simulink model "quadcopter_swarm_Perron_quaternion"  (R2023b)
settings: Solver=ode3  StartTime=0  StopTime=inf  FixedStep=0.005  RelTol=1e-3  EnableMultiTasking=on
values from neighbouring files (symbols this model uses):
  epsilon = 0.24975    [1nrx_dot.mat]    (also in 1nrxdrones_dot.mat; collision_avoidance_POS.mat; collision_avoidance_headonfix_POS.mat; collision_test.mat)
  F_e_g = [0 0 39.28]    [1nrx_dot.mat]    (also in 1nrxdrones_dot.mat; collision_avoidance_POS.mat; collision_avoidance_headonfix_POS.mat; collision_test.mat)
  g = 9.82    [1nrx_dot.mat]    (also in 1nrxdrones_dot.mat; collision_avoidance_POS.mat; collision_avoidance_headonfix_POS.mat; collision_test.mat)
  I_C = [0.5  0  0; 0  0.5  0; 0  0  1]    [1nrx_dot.mat]    (also in 1nrxdrones_dot.mat; collision_avoidance_POS.mat; collision_avoidance_headonfix_POS.mat; collision_test.mat)
  L = [4 -1 -1 -1 -1 0 -1 4 -1 -1 -1 0 ... (36 elements, 6x6)]    [1nrx_dot.mat]    (also in 1nrxdrones_dot.mat; collision_avoidance_POS.mat; collision_avoidance_headonfix_POS.mat; collision_test.mat)
  m = 4    [1nrx_dot.mat]    (also in 1nrxdrones_dot.mat; collision_avoidance_POS.mat; collision_avoidance_headonfix_POS.mat; collision_test.mat)
  M_RB = [4 0 0 0 0 0 0 4 0 0 0 0 ... (36 elements, 6x6)]    [1nrx_dot.mat]    (also in 1nrxdrones_dot.mat; collision_avoidance_POS.mat; collision_avoidance_headonfix_POS.mat; collision_test.mat)
  p_0 = [5  10; 5  -5; -8  5; 5  -13; 8  8; 0  0]    [1nrx_dot.mat]    (also in 1nrxdrones_dot.mat; collision_avoidance_POS.mat; collision_avoidance_headonfix_POS.mat; collision_test.mat)
  p_d = [1  0; 4  0; -2  0; 7  0; 9  0; 0  0]    [1nrx_dot.mat]    (also in 1nrxdrones_dot.mat; collision_avoidance_POS.mat; collision_avoidance_headonfix_POS.mat; collision_test.mat)
  V = [1 2 3 4 5 6]    [1nrx_dot.mat]    (also in 1nrxdrones_dot.mat; collision_avoidance_POS.mat; collision_avoidance_headonfix_POS.mat; collision_test.mat)
undefined symbols (not defined in the file or in its folder): PID_angle_max, PID_inner_max, PID_outer_max, PID_thrust_max
libraries: slpidlib x24, simulink_extras x20, dspsigops x15, sharedtransform x13, aerolibutil x11, dspindex x4, sharedutil x1, vrlib x1
(part 1 of 5)
settings Model: Creator=The MathWorks, Inc.  LastModifiedBy=frank
settings SolverCC: AlgebraicLoopSolver=TrustRegion
settings DataIOCC: LimitDataPoints=on  SaveFormat=Array  SaveOutput=off  SignalLogging=off  DSMLogging=off  SaveTime=off  ReturnWorkspaceOutputs=off
settings OptimizationCC: BlockReduction=off  BufferReuse=off  LifeSpan=inf
settings DebuggingCC: AlgebraicLoopMsg=none  ParameterPrecisionLossMsg=none  AllowSymbolicDim=off  PregeneratedLibrarySubsystemCodeDiagnostic=none  SFUnexpectedBacktrackingDiag=warning  SFNoUnconditionalDefaultTransitionDiag=warning  SFExecutionAtInitializationDiag=none  ArithmeticOperatorsInVariantConditions=warning
settings HardwareCC: ProdBitPerPointer=32  ProdBitPerSizeT=32  ProdBitPerPtrDiffT=32  ProdLargestAtomicFloat=None  ProdIntDivRoundTo=Undefined  ProdEndianess=Unspecified  ProdWordSize=32  ProdHWDeviceType=32-bit Generic
settings ModelReferenceCC: EnableRefExpFcnMdlSchedulingChecks=on  PropagateSignalLabelsOutOfModel=off
settings SFSimCC: SimUseLocalCustomCode=off  CustomCodeUndefinedFunction=UseInterfaceOnly
settings RTWCC: RTWUseLocalCustomCode=off  DLArmComputeVersion=19.05
settings CodeAppCC: StateflowObjectComments=on
settings GRTTargetCC: TargetLangStandard=C89/C90 (ANSI)
settings ConfigComp: CovMetricSettings=dw  CovSaveCumulativeToWorkspaceVar=on  CovSaveSingleToWorkspaceVar=on  CovExternalEMLEnable=off  CovSFcnEnable=off

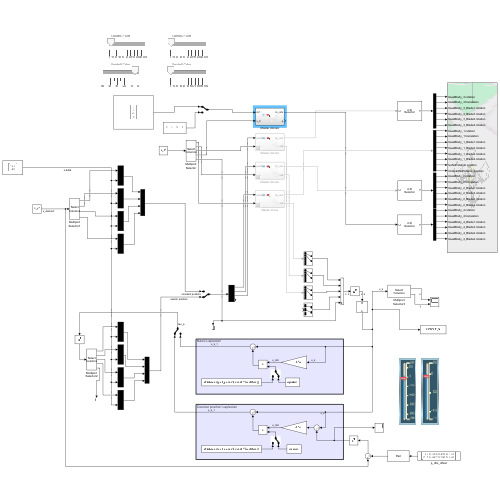
[thumbnail: Simulink's stored preview of the top-level diagram]
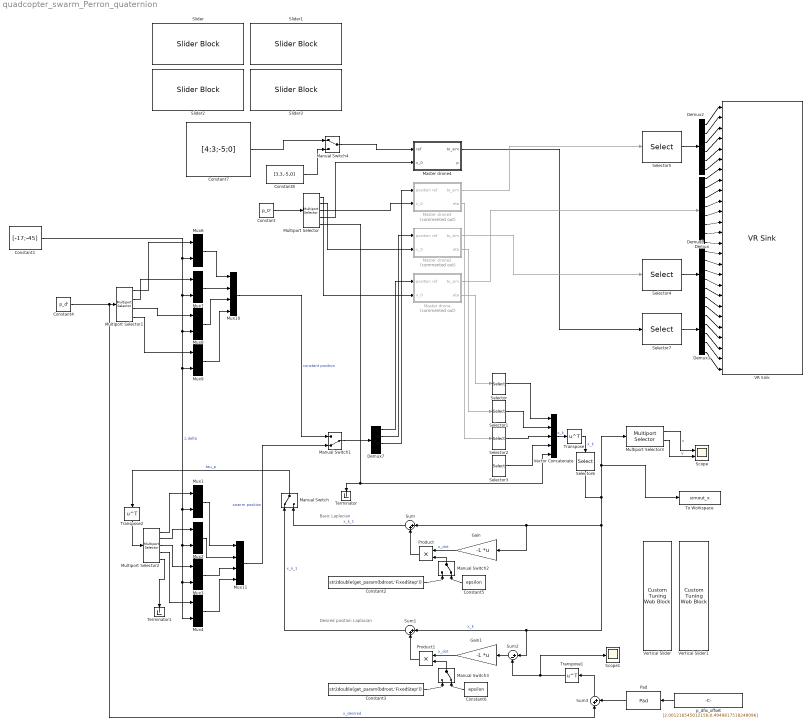
== system quadcopter_swarm_Perron_quaternion ==
  note: Basic Laplacian
  note: Desired position Laplacian
  Constant : Constant  Value=p_0'
  Constant1 : Constant  Value=[-17;-45]  VectorParams1D=off
  Constant2 : Constant  Value=str2double(get_param(bdroot,'FixedStep'))
  Constant3 : Constant  Value=str2double(get_param(bdroot,'FixedStep'))
  Constant4 : Constant  Value=p_d'
  Constant5 : Constant  Value=epsilon
  Constant6 : Constant  Value=epsilon
  Constant7 : Constant  Value=[4;3;-5;0]  VectorParams1D=off
  Constant8 : Constant  Value=[3,3,-5,0]
  Demux : Demux  Outputs=8
  Demux1 : Demux  Outputs=6
  Demux2 : Demux  Outputs=6
  Demux3 : Demux  Outputs=6
  Demux7 : Demux
  Gain : Gain  Gain=-L  Multiplication=Matrix(K*u)
  Gain1 : Gain  Gain=-L  Multiplication=Matrix(K*u)
  Manual Switch : ManualSwitch
  Manual Switch1 : ManualSwitch  CurrentSetting=0
  Manual Switch2 : ManualSwitch  CurrentSetting=0
  Manual Switch3 : ManualSwitch  CurrentSetting=0
  Manual Switch4 : ManualSwitch
  Master drone : Subsystem  Commented=on
  Master drone2 : Subsystem  Commented=on
  Master drone3 : Subsystem  Commented=on
  Master drone4 : Subsystem
  Multiport Selector : dspindex/Multiport Selector  rowsOrCols=Columns  idxCellArray={1,2,3,4,5}  idxErrMode=Clip Index
      settings: LibrarySourceBlock=|
      | dsphdlsupportsigmgmt/Multiport
      | Selector
  Multiport Selector1 : dspindex/Multiport Selector  rowsOrCols=Columns  idxCellArray={1,2,3,4}  idxErrMode=Clip Index
      settings: LibrarySourceBlock=|
      | dsphdlsupportsigmgmt/Multiport
      | Selector
  Multiport Selector2 : dspindex/Multiport Selector  rowsOrCols=Columns  idxCellArray={1,2,3,4,5}  idxErrMode=Clip Index
      settings: LibrarySourceBlock=|
      | dsphdlsupportsigmgmt/Multiport
      | Selector
  Multiport Selector3 : dspindex/Multiport Selector  rowsOrCols=Columns  idxCellArray={1,2}  idxErrMode=Clip Index
      settings: LibrarySourceBlock=|
      | dsphdlsupportsigmgmt/Multiport
      | Selector
  Mux{1..4,6..9} (8 alike) : Mux  Inputs=2
  Mux10 : Mux
  Mux11 : Mux
  Pad : dspsigops/Pad  padAlong=Rows  dimsToPad=1  valSrc=Specify via dialog  padVal=0  spec=Output size  padNumOutRowsSpecMethod=User-specified  numOutRows=2  padNumOutColsSpecMethod=User-specified  numOutCols=size(p_d,1)  isVarDimsMode=off  padBeginning=0  padEnd=0  outSizeMode=User-specified  outSize=1  padSigAt=Beginning  trunc_flag=None  roundingMode=Floor  overflowMode=off  truncOrWrapMode=Truncate  wrap_flag=None
  Product : Product
  Product1 : Product
  Scope : Scope  NumInputPorts=2
  Scope1 : Scope
  Selector : Selector  InputPortWidth=6  IndexOptions=Index vector (dialog)  Indices=1:2  OutputSizes=1
  Selector1 : Selector  InputPortWidth=6  IndexOptions=Index vector (dialog)  Indices=1:2  OutputSizes=1
  Selector2 : Selector  InputPortWidth=6  IndexOptions=Index vector (dialog)  Indices=1:2  OutputSizes=1
  Selector3 : Selector  InputPortWidth=3  IndexOptions=Index vector (dialog)  Indices=1:2  OutputSizes=1
  Selector4 : Selector  NumberOfDimensions=2  InputPortWidth=8  IndexOptions=Index vector (dialog),Select all  Indices=1:23,1  OutputSizes=1,1
  Selector5 : Selector  NumberOfDimensions=2  InputPortWidth=8  IndexOptions=Index vector (dialog),Select all  Indices=1:23,1  OutputSizes=1,1
  Selector6 : Selector  NumberOfDimensions=2  InputPortWidth=3  IndexOptions=Index vector (dialog),Select all  Indices=V,1  OutputSizes=1,1
  Selector7 : Selector  NumberOfDimensions=2  InputPortWidth=8  IndexOptions=Index vector (dialog),Select all  Indices=1:23,1  OutputSizes=1,1
  Slider : SliderBlock
  Slider1 : SliderBlock
  Slider2 : SliderBlock  ScaleMin=-50  ScaleMax=0
  Slider3 : SliderBlock
  Sum : Sum  Inputs=|++
  Sum1 : Sum  Inputs=|++
  Sum2 : Sum  Inputs=|+-
  Sum3 : Sum  Inputs=|++
  Terminator : Terminator
  Terminator1 : Terminator
  To Workspace : ToWorkspace  VariableName=simout_x  SampleTime=-1
      settings: Save2DSignal=2-D array (concatenate along first dimension)
  Transpose : Math  Operator=transpose
  Transpose1 : Math  Operator=transpose
  Transpose2 : Math  Operator=transpose
  VR Sink : vrlib/VR Sink  InstantiateOnLoad=on  SampleTime=12*0.005  ViewEnable=on  RemoteChange=off  RemoteView=off  FieldsWritten=QuadBody_3.rotation.4.1.1.double#QuadBody_3.translation.3.1.1.double#QuadBody_3_Blade1.rotation.4.1.1.double#QuadBody_3_Blade3.rotation.4.1.1.double#QuadBody_3_Blade2.rotation.4.1.1.double#QuadBody_3_Blade4.rotation.4.1.1.double#QuadBody_1.rotation.4.1.1.double#QuadBody_1.translation.3.1.1.double#QuadBody_1_Blade1.rotation.4.1.1.double#QuadBody_1_Blade3.rotation.4.1.1.double#QuadBody_1_Blade2.rotation.4.1.1.double#QuadBody_1_Blade4.rotation.4.1.1.double#IsoNoRotation.position.3.1.1.double#OnQuadNoRotation.position.3.1.1.double#QuadBody_2.rotation.4.1.1.double#QuadBody_2.translation.3.1.1.double#QuadBody_2_Blade1.rotation.4.1.1.double#QuadBody_2_Blade3.rotation.4.1.1.double#QuadBody_2_Blade2.rotation.4.1.1.double#QuadBody_2_Blade4.rotation.4.1.1.double#QuadBody_4.rotation.4.1.1.double#QuadBody_4.translation.3.1.1.double#QuadBody_4_Blade1.rotation.4.1.1.double#QuadBody_4_Blade3.rotation.4.1.1.double#QuadBody_4_Blade2.rotation.4.1.1.double#QuadBody_4_Blade4.rotation.4.1.1.double  WorldFileName=Quadcopter_VR.wrl  AutoView=on  VideoDimensions=[]  AllowVariableSize=off  FigureProperties="{'Position', 'Name', 'Viewpoint', 'CameraBound', 'CameraDirection', 'CameraPosition', 'CameraUpVector', 'ZoomFactor', 'Antialiasing', 'Headlight', 'Lighting', 'NavPanel', 'Sound', 'StatusBar', 'Stereo3D', 'Stereo3DCameraOffset', 'Stereo3DHIT', 'ToolBar', 'Textures', 'Transparency', 'Triad', 'Wireframe', 'NavZones', 'NavMode', 'NavSpeed', 'CaptureFileFormat', 'CaptureFileName', 'Record2DCompressMethod', 'Record2DCompressQuality', 'Record2D', 'Record2DFileName', 'Record2DFPS'; [2.0000000000000000e+00   8.4000000000000000e+01   8.6000000000000000e+02   5.6400000000000000e+02], '', 'Quad 4', 'on', [0.0000000000000000e+00   0.0000000000000000e+00  -1.0000000000000000e+00], [0.0000000000000000e+00   0.0000000000000000e+00   0.0000000000000000e+00], [0.0000000000000000e+00   1.0000000000000000e+00   0.0000000000000000e+00], [1.0000000000000000e+00], 'on', 'on', 'on', 'halfbar', 'on', 'on', 'off', [1.0000000149011612e-01], [0.0000000000000000e+00], 'on', 'on', 'on', 'none', 'off', 'off', 'examine', 'normal', 'tif', '%f_anim_%n.tif', 'auto', [7.5000000000000000e+01], 'off', '%f_anim_%n.avi', 'auto'}"
  Vector Concatenate : Concatenate  NumInputs=5  Mode=Multidimensional array  ConcatenateDimension=2
  Vertical Slider : CustomTuningWebBlock  LabelPosition=Hide  ShowInitialText=on  Configuration="{\"components\":[{\"name\":\"LinearScaleComponent\",\"settings\":{\"bounds\":{\"max\":30,\"min\":-90,\"tickInterval\":\"auto\"},\"internalTickHeightScaleFactor\":0.5,\"labelColor\":[255,255,200],\"labelFont\":{\"font\":\"Arial\",\"fontSize\":12},\"labelOffset\":0.05,\"labelTransparency\":1,\"needleImage\":{\"size\":[596,842],\"src\":\"data:image\\/svg+xml;base64,PD94bWwgdmVyc2lvbj0iMS4wIiBlbmNvZGluZz0idXRmLTgiPz4NCjwhLS0gR2VuZXJhdG9yOiBBZG9iZSBJbGx1c3RyYXRvciAyNS4wLjAsIFNWRyBFeHBvcnQgUGx1Zy1JbiAuIFNWRyBWZXJzaW9uOiA2LjAwIEJ1aWxkIDApICAtLT4NCjxzdmcgdmVyc2lvbj0iMS4xIg0KCSBpZD0ic3ZnOCIgeG1sbnM6Y2M9Imh0dHA6Ly9jcmVhdGl2ZWNvbW1vbnMub3JnL25zIyIgeG1sbnM6ZGM9Imh0dHA6Ly9wdXJsLm9yZy9kYy9lbGVtZW50cy8xLjEvIiB4bWxuczppbmtzY2FwZT0iaHR0cDovL3d3dy5pbmtzY2FwZS5vcmcvbmFtZXNw ...(+2420 chars)\",\"srcOrientation\":\"horizontal\"},\"needleOffset\":[0.0642123287671233,-0.8044596912521441],\"needleSize\":{\"height\":0.07668067226890757,\"width\":0.4337797619047619},\"position\":[0.03623949579831933,0.2829861111111111,0.6088789682539683,0.9196428571428571],\"referencePoint\":\"auto\",\"scaleColors\":[],\"scaleColorsSize\":0.2,\"scaleDirection\":\"BT\",\"showLabels\":1,\"showMinorTicks\":0,\"showSpanLine\":1,\"showTicks\":1,\"tickColor\":[252,252,197],\"tickTransparency\":1,\"valueBarColor\":[0,114,189],\"valueBarOffset\":-0.27,\"valueBarSize\":0.1,\"valueBarTransparency\":1}},{\"name\":\"BackgroundImageComponent\",\"settings\":{\"image\":{\"size\":[380,101],\"src\":\"data:image\\/svg+xml;base64,PHN2ZyB4bWxucz0iaHR0cDovL3d3dy53My5vcmcvMjAwMC9zdmciIHhtbG5zOnhsaW5rPSJodHRwOi8vd3d3LnczLm9yZy8xOTk5L3hsaW5rIiB2aWV3Qm94PSIwIDAgMzgwIDEwMSI+PGRlZnM+PHN0eWxlPi5jbHMtMXtmaWxsOiMwMDJiNDI7fS5jbHMtMntmaWxsOiM0MjcwODI7fS5jbHMtM3tmaWxsOnVybCgjcmFkaWFsLWdyYWRpZW50KTt9LmNscy00e2ZpbGw6I2M4YzhjODtzdHJva2U6IzAwMDt9PC9zdHlsZT48cmFkaWFsR3JhZGllbnQgaWQ9InJhZGlhbC1ncmFkaWVudCIgY3g9IjE5MCIgY3k9IjUwLjUiIHI9IjI2OS4yMSIgZ3JhZGllbnRVbml0cz0idXNlclNwYWNlT25Vc2UiPjxzdG9wIG9mZnNldD0iMC4wMSIgc3RvcC1jb2xvcj0iIzNlNGY1OCIvPjxzdG9wIG9mZnNldD0iMC4wNiIgc3RvcC1jb2xvcj0iIzQ0NTc2MSIvPjxzdG9wIG9mZnNldD0iMC4xNSIgc3RvcC1jb2xvcj0iIzU1NmE3NiIvPjxzdG9wIG9mZnNldD0iMC4yNSIgc3RvcC1jb2xvcj0iIzZkODg5NSIvPjxzdG9wIG9mZnNldD0iMC4zOCIgc3RvcC1jb2xvcj0iIzhmYjJjMyIvPjxzdG9wIG9mZnNldD0iMC41MiIgc3RvcC1jb2xvcj0iI2I2ZTRmYSIvPjxzdG9wIG9mZnNldD0iMSIgc3RvcC1jb2xvcj0iIzE1NDY1NyIvPjwvcmFkaWFsR3JhZGllbnQ+PC9kZWZzPjxnIGlkPSJmcmFtZSI+PGcgaWQ9IkxheWVyXzIiIGRhdGEtbmFtZT0iTGF5ZXIgMiI+PGcgaWQ9IkxheWVyXzEtMiIgZGF0YS1uYW1lPSJMYXllciAxLTIiPjxyZWN0IGlkPSJyZWN0MTAzNiIgY2xhc3M9ImNscy0xIiB4PSIxMSIgeT0iMTEiIHdpZHRoPSIzNTgiIGhlaWdodD0iNzkiLz48cGF0aCBpZD0icGF0aDEwMzgiIGNsYXNzPSJjbHMtMiIgZD0iTTgsOFY5M0gzNzJWOFpNMzY5LDkwSDExVjExSDM2OVoiLz48cGF0aCBpZD0icGF0aDEwNDAiIGNsYXNzPSJjbHMtMyIgZD0iTTAsMFYxMDFIMzgwVjBaTTM3Miw5M0g4VjhIMzcyWiIvPjwvZz48L2c+PC9nPjxnIGlkPSJ0cmFjayI+PHBhdGggaWQ9InJlY3QxNjExIiBjbGFzcz0iY2xzLTQiIGQ9Ik0zMy4zNywyNi41OUgzNDYuNjNjNCwwLDcuMjUsMi42LDcuMjUsNS44MWgwYzAsMy4yMS0zLjI1LDUuODItNy4yNSw1LjgySDMzLjM3Yy00LDAtNy4yNS0yLjYxLTcuMjUtNS44MmgwQzI2LjEyLDI5LjE5LDI5LjM3LDI2LjU5LDMzLjM3LDI2LjU5WiIvPjwvZz48L3N2Zz4=\",\"srcOrientation\":\"horizontal\"},\"position\":[0,0,1,1],\"scaleMode\":\"0\"}},{\"name\":\"ForegroundImageComponent\",\"settings\":{\"image\":{\"size\":[0,0],\"src\":\"default\",\"srcOrientation\":[]},\"isForeground\":1,\"position\":[0,0,1,1],\"scaleMode\":\"0\"}}],\"settings\":{\"BindingType\":\"param\",\"aspectRatio\":3.7777777777777777,\"backgroundColor\":[0,0,0,\"1\"],\"backgroundOffset\":0,\"backgroundOpacity\":1,\"fixedAspectRatio\":\"on\",\"foregroundColor\":[252,252,196],\"orientation\":\"vertical\",\"showBackgroundColor\":false,\"value\":0,\"version\":\"R2023a\"},\"type\":\"LinearGauge\"}"
  Vertical Slider1 : CustomTuningWebBlock  LabelPosition=Hide  ShowInitialText=on  Configuration="{\"components\":[{\"name\":\"LinearScaleComponent\",\"settings\":{\"bounds\":{\"max\":30,\"min\":-120,\"tickInterval\":\"auto\"},\"internalTickHeightScaleFactor\":0.5,\"labelColor\":[255,255,200],\"labelFont\":{\"font\":\"Arial\",\"fontSize\":12},\"labelOffset\":0.05,\"labelTransparency\":1,\"needleImage\":{\"size\":[596,842],\"src\":\"data:image\\/svg+xml;base64,PD94bWwgdmVyc2lvbj0iMS4wIiBlbmNvZGluZz0idXRmLTgiPz4NCjwhLS0gR2VuZXJhdG9yOiBBZG9iZSBJbGx1c3RyYXRvciAyNS4wLjAsIFNWRyBFeHBvcnQgUGx1Zy1JbiAuIFNWRyBWZXJzaW9uOiA2LjAwIEJ1aWxkIDApICAtLT4NCjxzdmcgdmVyc2lvbj0iMS4xIg0KCSBpZD0ic3ZnOCIgeG1sbnM6Y2M9Imh0dHA6Ly9jcmVhdGl2ZWNvbW1vbnMub3JnL25zIyIgeG1sbnM6ZGM9Imh0dHA6Ly9wdXJsLm9yZy9kYy9lbGVtZW50cy8xLjEvIiB4bWxuczppbmtzY2FwZT0iaHR0cDovL3d3dy5pbmtzY2FwZS5vcmcvbmFtZXNw ...(+2420 chars)\",\"srcOrientation\":\"horizontal\"},\"needleOffset\":[0.0642123287671233,-0.8044596912521441],\"needleSize\":{\"height\":0.07668067226890757,\"width\":0.4337797619047619},\"position\":[0.03623949579831933,0.2829861111111111,0.6088789682539683,0.9196428571428571],\"referencePoint\":\"auto\",\"scaleColors\":[],\"scaleColorsSize\":0.2,\"scaleDirection\":\"BT\",\"showLabels\":1,\"showMinorTicks\":0,\"showSpanLine\":1,\"showTicks\":1,\"tickColor\":[252,252,197],\"tickTransparency\":1,\"valueBarColor\":[0,114,189],\"valueBarOffset\":-0.27,\"valueBarSize\":0.1,\"valueBarTransparency\":1}},{\"name\":\"BackgroundImageComponent\",\"settings\":{\"image\":{\"size\":[380,101],\"src\":\"data:image\\/svg+xml;base64,PHN2ZyB4bWxucz0iaHR0cDovL3d3dy53My5vcmcvMjAwMC9zdmciIHhtbG5zOnhsaW5rPSJodHRwOi8vd3d3LnczLm9yZy8xOTk5L3hsaW5rIiB2aWV3Qm94PSIwIDAgMzgwIDEwMSI+PGRlZnM+PHN0eWxlPi5jbHMtMXtmaWxsOiMwMDJiNDI7fS5jbHMtMntmaWxsOiM0MjcwODI7fS5jbHMtM3tmaWxsOnVybCgjcmFkaWFsLWdyYWRpZW50KTt9LmNscy00e2ZpbGw6I2M4YzhjODtzdHJva2U6IzAwMDt9PC9zdHlsZT48cmFkaWFsR3JhZGllbnQgaWQ9InJhZGlhbC1ncmFkaWVudCIgY3g9IjE5MCIgY3k9IjUwLjUiIHI9IjI2OS4yMSIgZ3JhZGllbnRVbml0cz0idXNlclNwYWNlT25Vc2UiPjxzdG9wIG9mZnNldD0iMC4wMSIgc3RvcC1jb2xvcj0iIzNlNGY1OCIvPjxzdG9wIG9mZnNldD0iMC4wNiIgc3RvcC1jb2xvcj0iIzQ0NTc2MSIvPjxzdG9wIG9mZnNldD0iMC4xNSIgc3RvcC1jb2xvcj0iIzU1NmE3NiIvPjxzdG9wIG9mZnNldD0iMC4yNSIgc3RvcC1jb2xvcj0iIzZkODg5NSIvPjxzdG9wIG9mZnNldD0iMC4zOCIgc3RvcC1jb2xvcj0iIzhmYjJjMyIvPjxzdG9wIG9mZnNldD0iMC41MiIgc3RvcC1jb2xvcj0iI2I2ZTRmYSIvPjxzdG9wIG9mZnNldD0iMSIgc3RvcC1jb2xvcj0iIzE1NDY1NyIvPjwvcmFkaWFsR3JhZGllbnQ+PC9kZWZzPjxnIGlkPSJmcmFtZSI+PGcgaWQ9IkxheWVyXzIiIGRhdGEtbmFtZT0iTGF5ZXIgMiI+PGcgaWQ9IkxheWVyXzEtMiIgZGF0YS1uYW1lPSJMYXllciAxLTIiPjxyZWN0IGlkPSJyZWN0MTAzNiIgY2xhc3M9ImNscy0xIiB4PSIxMSIgeT0iMTEiIHdpZHRoPSIzNTgiIGhlaWdodD0iNzkiLz48cGF0aCBpZD0icGF0aDEwMzgiIGNsYXNzPSJjbHMtMiIgZD0iTTgsOFY5M0gzNzJWOFpNMzY5LDkwSDExVjExSDM2OVoiLz48cGF0aCBpZD0icGF0aDEwNDAiIGNsYXNzPSJjbHMtMyIgZD0iTTAsMFYxMDFIMzgwVjBaTTM3Miw5M0g4VjhIMzcyWiIvPjwvZz48L2c+PC9nPjxnIGlkPSJ0cmFjayI+PHBhdGggaWQ9InJlY3QxNjExIiBjbGFzcz0iY2xzLTQiIGQ9Ik0zMy4zNywyNi41OUgzNDYuNjNjNCwwLDcuMjUsMi42LDcuMjUsNS44MWgwYzAsMy4yMS0zLjI1LDUuODItNy4yNSw1LjgySDMzLjM3Yy00LDAtNy4yNS0yLjYxLTcuMjUtNS44MmgwQzI2LjEyLDI5LjE5LDI5LjM3LDI2LjU5LDMzLjM3LDI2LjU5WiIvPjwvZz48L3N2Zz4=\",\"srcOrientation\":\"horizontal\"},\"position\":[0,0,1,1],\"scaleMode\":\"0\"}},{\"name\":\"ForegroundImageComponent\",\"settings\":{\"image\":{\"size\":[0,0],\"src\":\"default\",\"srcOrientation\":[]},\"isForeground\":1,\"position\":[0,0,1,1],\"scaleMode\":\"0\"}}],\"settings\":{\"BindingType\":\"param\",\"aspectRatio\":3.7777777777777777,\"backgroundColor\":[0,0,0,\"1\"],\"backgroundOffset\":0,\"backgroundOpacity\":1,\"fixedAspectRatio\":\"on\",\"foregroundColor\":[252,252,196],\"orientation\":\"vertical\",\"showBackgroundColor\":false,\"value\":0,\"version\":\"R2023a\"},\"type\":\"LinearGauge\"}"
  p_dfix_offset : Constant  Value=[2.001216545012156;0.4949817518248096]  VectorParams1D=off
  wires:
  Demux/1 -> VR Sink/7
  Demux/2 -> VR Sink/8
  Demux/3 -> VR Sink/9
  Demux/4 -> VR Sink/10
  Demux/5 -> VR Sink/11
  Demux/6 -> VR Sink/12
  Demux1/1 -> VR Sink/15
  Demux1/2 -> VR Sink/16
  Demux1/3 -> VR Sink/17
  Demux1/4 -> VR Sink/18
  Demux1/5 -> VR Sink/19
  Demux1/6 -> VR Sink/20
  Demux3/1 -> VR Sink/21
  Demux3/2 -> VR Sink/22
  Demux3/3 -> VR Sink/23
  Demux3/4 -> VR Sink/24
  Demux3/5 -> VR Sink/25
  Demux3/6 -> VR Sink/26
  Demux2/6 -> VR Sink/6
  Demux2/5 -> VR Sink/5
  Demux2/4 -> VR Sink/4
  Demux2/3 -> VR Sink/3
  Demux2/2 -> VR Sink/2
  Demux2/1 -> VR Sink/1
  Selector5/1 -> Demux2/1
  Selector7/1 -> Demux3/1
  Selector4/1 -> Demux1/1
  Demux/7 -> VR Sink/13
  Demux/8 -> VR Sink/14
  Master drone/2(eta) -> Selector/1
  Master drone2/2(eta) -> Selector1/1
  Master drone3/2(eta) -> Selector2/1
  Selector/1 -> Vector Concatenate/1
  Selector1/1 -> Vector Concatenate/2
  Selector2/1 -> Vector Concatenate/3
  Selector3/1 -> Vector Concatenate/4
  Multiport Selector/1 -> Master drone/2(x_0)
  Multiport Selector/2 -> Master drone2/2(x_0)
  Multiport Selector/3 -> Master drone3/2(x_0)
  Multiport Selector/4 -> Master drone4/2(x_0)
  Sum/1 -> Manual Switch/2  "x_k_1"
  Demux7/1 -> Master drone/1(position ref)
  Multiport Selector2/1 -> Mux1/1
  Multiport Selector2/2 -> Mux2/1
  Demux7/2 -> Master drone2/1(position ref)
  Multiport Selector2/3 -> Mux3/1
  Multiport Selector2/4 -> Mux4/1
  Demux7/3 -> Master drone3/1(position ref)
  Gain/1 -> Product/1  "x_dot"
  Constant2/1 -> Manual Switch2/1
  Product/1 -> Sum/2
  Product1/1 -> Sum1/2
  Sum1/1 -> Manual Switch/1  "x_k_1"
  Gain1/1 -> Product1/1  "x_dot"
  Selector6/1 -> Multiport Selector3/1, To Workspace/1, Sum2/1, Sum1/1, Sum/1, Gain/1  "x_k"
  Manual Switch/1 -> Transpose2/1  "tau_p"
  Constant1/1 -> Mux4/2, Mux3/2, Mux2/2, Mux1/2, Mux9/2, Mux8/2, Mux7/2, Mux6/2  "z,delta"
  Mux6/1 -> Mux10/1
  Mux7/1 -> Mux10/2
  Mux8/1 -> Mux10/3
  Mux9/1 -> Mux10/4
  Manual Switch1/1 -> Demux7/1
  Mux11/1 -> Manual Switch1/2  "swarm position"
  Mux10/1 -> Manual Switch1/1  "constant position"
  Mux1/1 -> Mux11/1
  Mux2/1 -> Mux11/2
  Mux3/1 -> Mux11/3
  Mux4/1 -> Mux11/4
  Constant4/1 -> Sum3/1, Multiport Selector1/1  "x_desired"
  Multiport Selector1/1 -> Mux6/1
  Multiport Selector1/2 -> Mux7/1
  Multiport Selector1/3 -> Mux8/1
  Multiport Selector1/4 -> Mux9/1
  Constant5/1 -> Manual Switch2/2
  Manual Switch2/1 -> Product/2
  Sum2/1 -> Gain1/1
  Constant6/1 -> Manual Switch3/2
  Constant3/1 -> Manual Switch3/1
  Manual Switch3/1 -> Product1/2
  Sum3/1 -> Transpose1/1
  Constant/1 -> Multiport Selector/1
  p_dfix_offset/1 -> Pad/1
  Pad/1 -> Sum3/2
  Vector Concatenate/1 -> Transpose/1  "x_k"
  Transpose1/1 -> Scope1/1, Sum2/2
  Transpose2/1 -> Multiport Selector2/1
  Multiport Selector3/1 -> Scope/1  "x"
  Multiport Selector3/2 -> Scope/2  "y"
  Transpose/1 -> Selector6/1  "x_k"
  Multiport Selector/5 -> Terminator/1, Vector Concatenate/5
  Multiport Selector2/5 -> Terminator1/1
  Constant7/1 -> Manual Switch4/1
  Constant8/1 -> Manual Switch4/2
  Manual Switch4/1 -> Master drone4/1(ref)
  Master drone4/1(to_sim) -> Selector7/1
  Master drone3/1(to_sim) -> Selector5/1
  Master drone2/1(to_sim) -> Selector4/1
  Master drone/1(to_sim) -> Demux/1

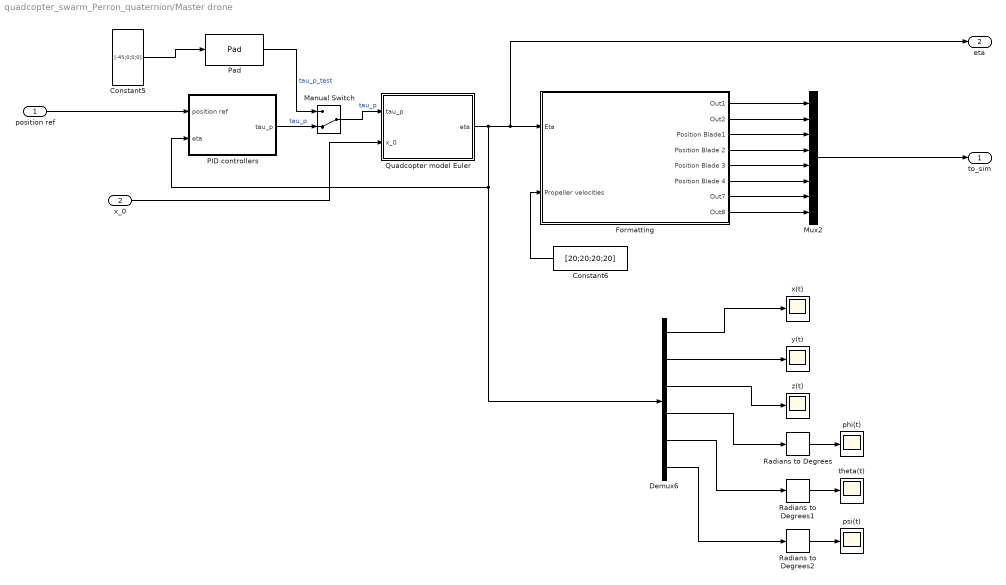
== system quadcopter_swarm_Perron_quaternion/Master drone ==
  position ref : Inport
  x_0 : Inport  Port=2
  Constant5 : Constant  Value=[-45;0;0;0]  VectorParams1D=off
  Constant6 : Constant  Value=[20;20;20;20]  VectorParams1D=off
  Demux6 : Demux  Outputs=6
  Formatting : Subsystem
  Manual Switch : ManualSwitch  CurrentSetting=0
  Mux2 : Mux  Inputs=8
  PID controllers : Subsystem
  Pad : dspsigops/Pad  padAlong=Specified dimensions  dimsToPad=1  valSrc=Specify via dialog  padVal=0  spec=Output size  padNumOutRowsSpecMethod=User-specified  numOutRows=1  padNumOutColsSpecMethod=User-specified  numOutCols=6  isVarDimsMode=off  padBeginning=0  padEnd=0  outSizeMode=User-specified  outSize=6  padSigAt=Beginning  trunc_flag=None  roundingMode=Floor  overflowMode=off  truncOrWrapMode=Truncate  wrap_flag=None
  Quadcopter model Euler : Subsystem
  Radians to Degrees : simulink_extras/Transformations/Radians to Degrees
  Radians to Degrees1 : simulink_extras/Transformations/Radians to Degrees
  Radians to Degrees2 : simulink_extras/Transformations/Radians to Degrees
  phi(t) : Scope
  psi(t) : Scope
  theta(t) : Scope
  x(t) : Scope
  y(t) : Scope
  z(t) : Scope
  to_sim : Outport
  eta : Outport  Port=2
  wires:
  Formatting/6(Position Blade 4) -> Mux2/6
  Demux6/1 -> x(t)/1
  Demux6/6 -> Radians to Degrees2/1
  Manual Switch/1 -> Quadcopter model Euler/1(tau_p)  "tau_p"
  Pad/1 -> Manual Switch/1  "tau_p_test"
  Radians to Degrees2/1 -> psi(t)/1
  Demux6/5 -> Radians to Degrees1/1
  Formatting/3(Position Blade1) -> Mux2/3
  Formatting/2(Out2) -> Mux2/2
  Demux6/4 -> Radians to Degrees/1
  position ref/1 -> PID controllers/1(position ref)
  Demux6/3 -> z(t)/1
  Constant6/1 -> Formatting/2(Propeller velocities)
  Constant5/1 -> Pad/1
  Demux6/2 -> y(t)/1
  Formatting/7(Out7) -> Mux2/7
  Radians to Degrees1/1 -> theta(t)/1
  Formatting/8(Out8) -> Mux2/8
  Radians to Degrees/1 -> phi(t)/1
  Formatting/5(Position Blade 3) -> Mux2/5
  Formatting/4(Position Blade 2) -> Mux2/4
  Formatting/1(Out1) -> Mux2/1
  PID controllers/1(tau_p) -> Manual Switch/2  "tau_p"
  Mux2/1 -> to_sim/1
  Quadcopter model Euler/1(eta) -> Demux6/1, PID controllers/2(eta), eta/1, Formatting/1(Eta)
  x_0/1 -> Quadcopter model Euler/2(x_0)

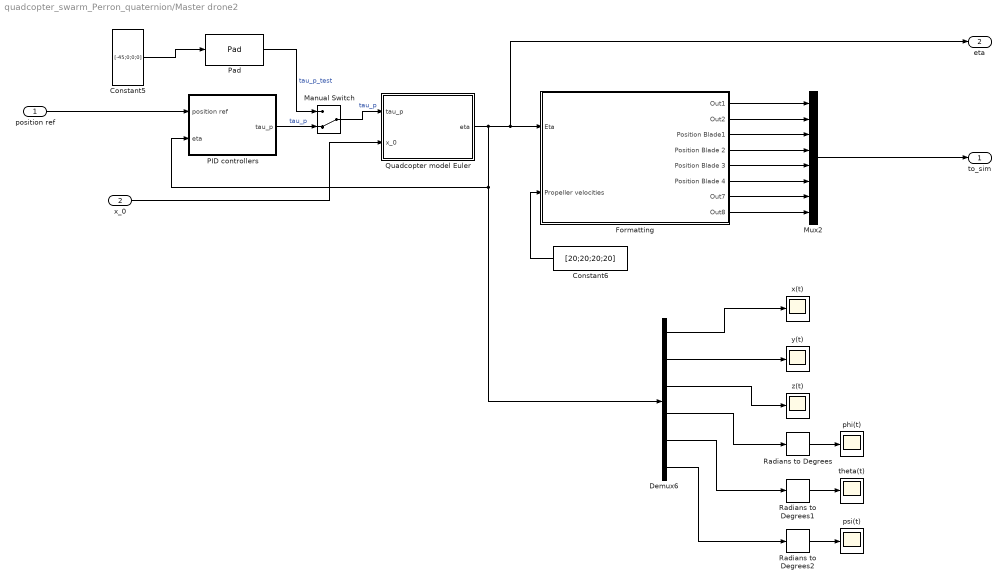
== system quadcopter_swarm_Perron_quaternion/Master drone2 ==
  position ref : Inport
  x_0 : Inport  Port=2
  Constant5 : Constant  Value=[-45;0;0;0]  VectorParams1D=off
  Constant6 : Constant  Value=[20;20;20;20]  VectorParams1D=off
  Demux6 : Demux  Outputs=6
  Formatting : Subsystem
  Manual Switch : ManualSwitch  CurrentSetting=0
  Mux2 : Mux  Inputs=8
  PID controllers : Subsystem
  Pad : dspsigops/Pad  padAlong=Specified dimensions  dimsToPad=1  valSrc=Specify via dialog  padVal=0  spec=Output size  padNumOutRowsSpecMethod=User-specified  numOutRows=1  padNumOutColsSpecMethod=User-specified  numOutCols=6  isVarDimsMode=off  padBeginning=0  padEnd=0  outSizeMode=User-specified  outSize=6  padSigAt=Beginning  trunc_flag=None  roundingMode=Floor  overflowMode=off  truncOrWrapMode=Truncate  wrap_flag=None
  Quadcopter model Euler : Subsystem
  Radians to Degrees : simulink_extras/Transformations/Radians to Degrees
  Radians to Degrees1 : simulink_extras/Transformations/Radians to Degrees
  Radians to Degrees2 : simulink_extras/Transformations/Radians to Degrees
  phi(t) : Scope
  psi(t) : Scope
  theta(t) : Scope
  x(t) : Scope
  y(t) : Scope
  z(t) : Scope
  to_sim : Outport
  eta : Outport  Port=2
  wires:
  Formatting/6(Position Blade 4) -> Mux2/6
  Demux6/1 -> x(t)/1
  Demux6/6 -> Radians to Degrees2/1
  Manual Switch/1 -> Quadcopter model Euler/1(tau_p)  "tau_p"
  Pad/1 -> Manual Switch/1  "tau_p_test"
  Radians to Degrees2/1 -> psi(t)/1
  Demux6/5 -> Radians to Degrees1/1
  Formatting/3(Position Blade1) -> Mux2/3
  Formatting/2(Out2) -> Mux2/2
  Demux6/4 -> Radians to Degrees/1
  position ref/1 -> PID controllers/1(position ref)
  Demux6/3 -> z(t)/1
  Constant6/1 -> Formatting/2(Propeller velocities)
  Constant5/1 -> Pad/1
  Demux6/2 -> y(t)/1
  Formatting/7(Out7) -> Mux2/7
  Radians to Degrees1/1 -> theta(t)/1
  Formatting/8(Out8) -> Mux2/8
  Radians to Degrees/1 -> phi(t)/1
  Formatting/5(Position Blade 3) -> Mux2/5
  Formatting/4(Position Blade 2) -> Mux2/4
  Formatting/1(Out1) -> Mux2/1
  PID controllers/1(tau_p) -> Manual Switch/2  "tau_p"
  Mux2/1 -> to_sim/1
  Quadcopter model Euler/1(eta) -> Demux6/1, PID controllers/2(eta), eta/1, Formatting/1(Eta)
  x_0/1 -> Quadcopter model Euler/2(x_0)

== system quadcopter_swarm_Perron_quaternion/Master drone3 ==
  position ref : Inport
  x_0 : Inport  Port=2
  Constant5 : Constant  Value=[-45;0;0;0]  VectorParams1D=off
  Constant6 : Constant  Value=[20;20;20;20]  VectorParams1D=off
  Demux6 : Demux  Outputs=6
  Formatting : Subsystem
  Manual Switch : ManualSwitch  CurrentSetting=0
  Mux2 : Mux  Inputs=8
  PID controllers : Subsystem
  Pad : dspsigops/Pad  padAlong=Specified dimensions  dimsToPad=1  valSrc=Specify via dialog  padVal=0  spec=Output size  padNumOutRowsSpecMethod=User-specified  numOutRows=1  padNumOutColsSpecMethod=User-specified  numOutCols=6  isVarDimsMode=off  padBeginning=0  padEnd=0  outSizeMode=User-specified  outSize=6  padSigAt=Beginning  trunc_flag=None  roundingMode=Floor  overflowMode=off  truncOrWrapMode=Truncate  wrap_flag=None
  Quadcopter model Euler : Subsystem
  Radians to Degrees : simulink_extras/Transformations/Radians to Degrees
  Radians to Degrees1 : simulink_extras/Transformations/Radians to Degrees
  Radians to Degrees2 : simulink_extras/Transformations/Radians to Degrees
  phi(t) : Scope
  psi(t) : Scope
  theta(t) : Scope
  x(t) : Scope
  y(t) : Scope
  z(t) : Scope
  to_sim : Outport
  eta : Outport  Port=2
  wires:
  Formatting/6(Position Blade 4) -> Mux2/6
  Demux6/1 -> x(t)/1
  Demux6/6 -> Radians to Degrees2/1
  Manual Switch/1 -> Quadcopter model Euler/1(tau_p)  "tau_p"
  Pad/1 -> Manual Switch/1  "tau_p_test"
  Radians to Degrees2/1 -> psi(t)/1
  Demux6/5 -> Radians to Degrees1/1
  Formatting/3(Position Blade1) -> Mux2/3
  Formatting/2(Out2) -> Mux2/2
  Demux6/4 -> Radians to Degrees/1
  position ref/1 -> PID controllers/1(position ref)
  Demux6/3 -> z(t)/1
  Constant6/1 -> Formatting/2(Propeller velocities)
  Constant5/1 -> Pad/1
  Demux6/2 -> y(t)/1
  Formatting/7(Out7) -> Mux2/7
  Radians to Degrees1/1 -> theta(t)/1
  Formatting/8(Out8) -> Mux2/8
  Radians to Degrees/1 -> phi(t)/1
  Formatting/5(Position Blade 3) -> Mux2/5
  Formatting/4(Position Blade 2) -> Mux2/4
  Formatting/1(Out1) -> Mux2/1
  PID controllers/1(tau_p) -> Manual Switch/2  "tau_p"
  Mux2/1 -> to_sim/1
  Quadcopter model Euler/1(eta) -> Demux6/1, PID controllers/2(eta), eta/1, Formatting/1(Eta)
  x_0/1 -> Quadcopter model Euler/2(x_0)

== system quadcopter_swarm_Perron_quaternion/Master drone4 ==
  ref : Inport
  x_0 : Inport  Port=2
  Constant1 : Constant  Value=[-g*m;1;0;0]  VectorParams1D=off
  Constant5 : Constant  Value=[-g*m;0;0;0]  VectorParams1D=off
  Constant6 : Constant  Value=[20;20;20;20]  VectorParams1D=off
  Formatting : Subsystem
  Manual Switch : ManualSwitch
  Manual Switch1 : ManualSwitch  CurrentSetting=0
  Mux2 : Mux  Inputs=8
  PID controllers : Subsystem
  Pad : dspsigops/Pad  padAlong=Specified dimensions  dimsToPad=1  valSrc=Specify via dialog  padVal=0  spec=Output size  padNumOutRowsSpecMethod=User-specified  numOutRows=1  padNumOutColsSpecMethod=User-specified  numOutCols=6  isVarDimsMode=off  padBeginning=0  padEnd=0  outSizeMode=User-specified  outSize=6  padSigAt=Beginning  trunc_flag=None  roundingMode=Floor  overflowMode=off  truncOrWrapMode=Truncate  wrap_flag=None
  Quadcopter model : Subsystem
  Quaternions to Rotation Angles : sharedtransform/Quaternions to Rotation Angles  rotationOrder=XYZ  aMode=aMode
  Radians to Degrees : simulink_extras/Transformations/Radians to Degrees
  Radians to Degrees1 : simulink_extras/Transformations/Radians to Degrees
  odometry : Scope  NumInputPorts=3
  q to Theta_b_b_e : Subsystem
  to_sim : Outport
  p : Outport  Port=2
  wires:
  Formatting/6(Position Blade 4) -> Mux2/6
  Manual Switch/1 -> Quadcopter model/1(tau_p)  "tau_p_b"
  Pad/1 -> Manual Switch/1  "tau_p_test"
  Formatting/3(Position Blade1) -> Mux2/3
  Formatting/2(Out2) -> Mux2/2
  ref/1 -> PID controllers/1(ref)
  Constant6/1 -> Formatting/3(Propeller velocities)
  Constant5/1 -> Manual Switch1/2
  Formatting/7(Out7) -> Mux2/7
  Formatting/8(Out8) -> Mux2/8
  Radians to Degrees/1 -> odometry/2  "Theta_b_b_e"
  Formatting/5(Position Blade 3) -> Mux2/5
  Formatting/4(Position Blade 2) -> Mux2/4
  Formatting/1(Out1) -> Mux2/1
  PID controllers/1(tau_p_b) -> Manual Switch/2  "tau_p"
  Mux2/1 -> to_sim/1
  x_0/1 -> Quadcopter model/2(p_0)
  Quadcopter model/1(p) -> PID controllers/2(p), p/1, odometry/1, Formatting/1(p)  "p_e_b_e"
  Quadcopter model/2(q) -> q to Theta_b_b_e/1(q), Quaternions to Rotation Angles/1, PID controllers/3(q), Formatting/2(q)
  Constant1/1 -> Manual Switch1/1
  Manual Switch1/1 -> Pad/1
  Quaternions to Rotation Angles/1 -> Radians to Degrees/1  "Theta_b_b_e"
  q to Theta_b_b_e/1(Theta_b_b_e) -> Radians to Degrees1/1
  Radians to Degrees1/1 -> odometry/3  "Theta_b_b_e"

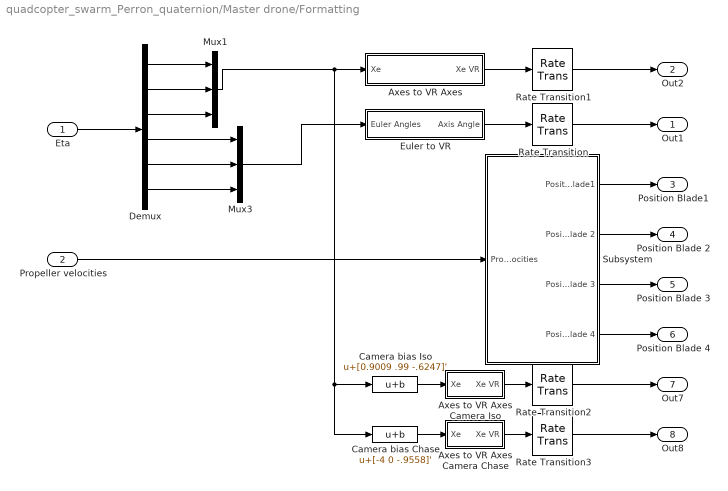
== system quadcopter_swarm_Perron_quaternion/Master drone/Formatting ==
  Eta : Inport
  Propeller velocities : Inport  Port=2
  Axes to VR Axes : Subsystem
  Axes to VR Axes Camera Chase : Subsystem
  Axes to VR Axes Camera Iso : Subsystem
  Camera bias Chase : Bias  Bias=[-4 0 -.9558]'  SaturateOnIntegerOverflow=off
  Camera bias Iso : Bias  Bias=[0.9009 .99 -.6247]'  SaturateOnIntegerOverflow=off
  Demux : Demux  Outputs=6
  Euler to VR : Subsystem
  Mux1 : Mux  Inputs=3
  Mux3 : Mux  Inputs=3
  Rate Transition{,1..3} (4 alike) : RateTransition
  Subsystem : Subsystem
  Out1 : Outport
  Out2 : Outport  Port=2
  Position Blade1 : Outport  Port=3
  Position Blade 2 : Outport  Port=4
  Position Blade 3 : Outport  Port=5
  Position Blade 4 : Outport  Port=6
  Out7 : Outport  Port=7
  Out8 : Outport  Port=8
  wires:
  Rate Transition2/1 -> Out7/1
  Propeller velocities/1 -> Subsystem/1(Propeller velocities)
  Subsystem/3(Position Blade 3) -> Position Blade 3/1
  Subsystem/1(Position Blade1) -> Position Blade1/1
  Mux3/1 -> Euler to VR/1(Euler Angles)
  Camera bias Chase/1 -> Axes to VR Axes Camera Chase/1(Xe)
  Axes to VR Axes Camera Chase/1(Xe VR) -> Rate Transition3/1
  Subsystem/2(Position Blade 2) -> Position Blade 2/1
  Axes to VR Axes Camera Iso/1(Xe VR) -> Rate Transition2/1
  Euler to VR/1(Axis Angle) -> Rate Transition/1
  Axes to VR Axes/1(Xe VR) -> Rate Transition1/1
  Rate Transition1/1 -> Out2/1
  Camera bias Iso/1 -> Axes to VR Axes Camera Iso/1(Xe)
  Mux1/1 -> Camera bias Chase/1, Camera bias Iso/1, Axes to VR Axes/1(Xe)
  Rate Transition3/1 -> Out8/1
  Rate Transition/1 -> Out1/1
  Subsystem/4(Position Blade 4) -> Position Blade 4/1
  Demux/2 -> Mux1/2
  Demux/5 -> Mux3/2
  Demux/3 -> Mux1/3
  Eta/1 -> Demux/1
  Demux/1 -> Mux1/1
  Demux/4 -> Mux3/1
  Demux/6 -> Mux3/3

== system quadcopter_swarm_Perron_quaternion/Master drone/PID controllers ==
  position ref : Inport
  eta : Inport  Port=2
  Inner-loop controllers : Subsystem
  Manual Switch : ManualSwitch
  Pad3 : dspsigops/Pad  padAlong=Rows  dimsToPad=1  valSrc=Specify via dialog  padVal=0  spec=Output size  padNumOutRowsSpecMethod=User-specified  numOutRows=1  padNumOutColsSpecMethod=User-specified  numOutCols=6  isVarDimsMode=off  padBeginning=0  padEnd=0  outSizeMode=User-specified  outSize=1  padSigAt=Beginning  trunc_flag=None  roundingMode=Floor  overflowMode=off  truncOrWrapMode=Truncate  wrap_flag=None
  Refs (alt. + Euler angles) : Constant  Value=[-20;0;20;0]  VectorParams1D=off
  outer-loop controllers output : Scope
  outer-loop position controller : Subsystem
  tau_p : Outport
  wires:
  position ref/1 -> outer-loop position controller/1(position ref)
  outer-loop position controller/1(alt. + Euler angles) -> Manual Switch/1, outer-loop controllers output/1
  eta/1 -> Inner-loop controllers/2(eta), outer-loop position controller/2(eta_euler)  "eta_euler"
  Refs (alt. + Euler angles)/1 -> Manual Switch/2
  Manual Switch/1 -> Inner-loop controllers/1(refs)  "alt. + Euler angles"
  Pad3/1 -> tau_p/1
  Inner-loop controllers/1(Fz,mx,my,mz) -> Pad3/1

== system quadcopter_swarm_Perron_quaternion/Master drone/Quadcopter model Euler ==
  tau_p : Inport
  x_0 : Inport  Port=2
  Gravity : Subsystem
      settings: PortSchema="{\"entries\":[{\"content\":{\"sides\":[{\"content\":{\"connectorIds\":[\"Out1\",\"In1\"]},\"type\":\"ConnectorPlacement.EquallySpacedRectSide\",\"uuid\":\"bc23a1f5-cdb9-4283-9ea4-cdee480fdcbc\"},{\"content\":{\"side\":\"RIGHT\"},\"type\":\"ConnectorPlacement.EquallySpacedRectSide\",\"uuid\":\"6d80009b-5037-4ff5-9c53-c950dec4dc37\"},{\"content\":{\"side\":\"TOP\"},\"type\":\"ConnectorPlacement.EquallySpacedRectSide\",\"uuid\":\"00364382-26ff-4cd9-a2a2-07aec872e2b0\"}]},\"type\":\"ConnectorPlacement.EquallySpacedConnector\",\"uuid\":\"88fcb791-5b95-44c0-bf21-2ced4fb8e0fb\"}],\"packageUris\":[\"http://schema.mathworks.com/mf0/Connector/R2020b\"],\"version\":\"1.0\"}"
  Scope1 : Scope  NumInputPorts=3
  Sum : Sum  Inputs=|++
  kinematics from Euler angles : Subsystem
  rigid-body dynamics : Subsystem
  eta : Outport
  wires:
  kinematics from Euler angles/1(eta) -> eta/1, Gravity/1(eta_euler), Scope1/3
  tau_p/1 -> Sum/1  "tau_p"
  Sum/1 -> Scope1/1, rigid-body dynamics/1(tau)  "tau"
  rigid-body dynamics/1(nu_subsystem) -> Scope1/2, kinematics from Euler angles/1(nu)
  Gravity/1(tau_g) -> Sum/2
  x_0/1 -> kinematics from Euler angles/2(x_0)

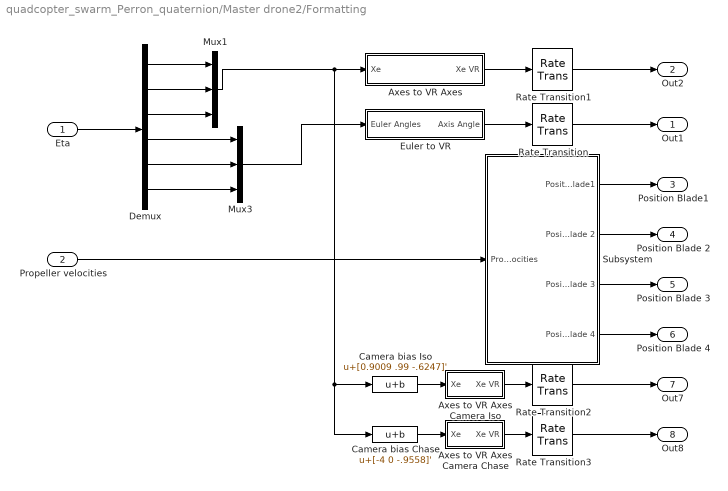
== system quadcopter_swarm_Perron_quaternion/Master drone2/Formatting ==
  Eta : Inport
  Propeller velocities : Inport  Port=2
  Axes to VR Axes : Subsystem
  Axes to VR Axes Camera Chase : Subsystem
  Axes to VR Axes Camera Iso : Subsystem
  Camera bias Chase : Bias  Bias=[-4 0 -.9558]'  SaturateOnIntegerOverflow=off
  Camera bias Iso : Bias  Bias=[0.9009 .99 -.6247]'  SaturateOnIntegerOverflow=off
  Demux : Demux  Outputs=6
  Euler to VR : Subsystem
  Mux1 : Mux  Inputs=3
  Mux3 : Mux  Inputs=3
  Rate Transition{,1..3} (4 alike) : RateTransition
  Subsystem : Subsystem
  Out1 : Outport
  Out2 : Outport  Port=2
  Position Blade1 : Outport  Port=3
  Position Blade 2 : Outport  Port=4
  Position Blade 3 : Outport  Port=5
  Position Blade 4 : Outport  Port=6
  Out7 : Outport  Port=7
  Out8 : Outport  Port=8
  wires:
  Rate Transition2/1 -> Out7/1
  Propeller velocities/1 -> Subsystem/1(Propeller velocities)
  Subsystem/3(Position Blade 3) -> Position Blade 3/1
  Subsystem/1(Position Blade1) -> Position Blade1/1
  Mux3/1 -> Euler to VR/1(Euler Angles)
  Camera bias Chase/1 -> Axes to VR Axes Camera Chase/1(Xe)
  Axes to VR Axes Camera Chase/1(Xe VR) -> Rate Transition3/1
  Subsystem/2(Position Blade 2) -> Position Blade 2/1
  Axes to VR Axes Camera Iso/1(Xe VR) -> Rate Transition2/1
  Euler to VR/1(Axis Angle) -> Rate Transition/1
  Axes to VR Axes/1(Xe VR) -> Rate Transition1/1
  Rate Transition1/1 -> Out2/1
  Camera bias Iso/1 -> Axes to VR Axes Camera Iso/1(Xe)
  Mux1/1 -> Camera bias Chase/1, Camera bias Iso/1, Axes to VR Axes/1(Xe)
  Rate Transition3/1 -> Out8/1
  Rate Transition/1 -> Out1/1
  Subsystem/4(Position Blade 4) -> Position Blade 4/1
  Demux/2 -> Mux1/2
  Demux/5 -> Mux3/2
  Demux/3 -> Mux1/3
  Eta/1 -> Demux/1
  Demux/1 -> Mux1/1
  Demux/4 -> Mux3/1
  Demux/6 -> Mux3/3

== system quadcopter_swarm_Perron_quaternion/Master drone2/PID controllers ==
  position ref : Inport
  eta : Inport  Port=2
  Inner-loop controllers : Subsystem
  Manual Switch : ManualSwitch
  Pad3 : dspsigops/Pad  padAlong=Rows  dimsToPad=1  valSrc=Specify via dialog  padVal=0  spec=Output size  padNumOutRowsSpecMethod=User-specified  numOutRows=1  padNumOutColsSpecMethod=User-specified  numOutCols=6  isVarDimsMode=off  padBeginning=0  padEnd=0  outSizeMode=User-specified  outSize=1  padSigAt=Beginning  trunc_flag=None  roundingMode=Floor  overflowMode=off  truncOrWrapMode=Truncate  wrap_flag=None
  Refs (alt. + Euler angles) : Constant  Value=[-20;0;20;0]  VectorParams1D=off
  outer-loop controllers output : Scope
  outer-loop position controller : Subsystem
  tau_p : Outport
  wires:
  position ref/1 -> outer-loop position controller/1(position ref)
  outer-loop position controller/1(alt. + Euler angles) -> Manual Switch/1, outer-loop controllers output/1
  eta/1 -> Inner-loop controllers/2(eta), outer-loop position controller/2(eta_euler)  "eta_euler"
  Refs (alt. + Euler angles)/1 -> Manual Switch/2
  Manual Switch/1 -> Inner-loop controllers/1(refs)  "alt. + Euler angles"
  Pad3/1 -> tau_p/1
  Inner-loop controllers/1(Fz,mx,my,mz) -> Pad3/1

== system quadcopter_swarm_Perron_quaternion/Master drone2/Quadcopter model Euler ==
  tau_p : Inport
  x_0 : Inport  Port=2
  Gravity : Subsystem
      settings: PortSchema="{\"entries\":[{\"content\":{\"sides\":[{\"content\":{\"connectorIds\":[\"Out1\",\"In1\"]},\"type\":\"ConnectorPlacement.EquallySpacedRectSide\",\"uuid\":\"bc23a1f5-cdb9-4283-9ea4-cdee480fdcbc\"},{\"content\":{\"side\":\"RIGHT\"},\"type\":\"ConnectorPlacement.EquallySpacedRectSide\",\"uuid\":\"6d80009b-5037-4ff5-9c53-c950dec4dc37\"},{\"content\":{\"side\":\"TOP\"},\"type\":\"ConnectorPlacement.EquallySpacedRectSide\",\"uuid\":\"00364382-26ff-4cd9-a2a2-07aec872e2b0\"}]},\"type\":\"ConnectorPlacement.EquallySpacedConnector\",\"uuid\":\"88fcb791-5b95-44c0-bf21-2ced4fb8e0fb\"}],\"packageUris\":[\"http://schema.mathworks.com/mf0/Connector/R2020b\"],\"version\":\"1.0\"}"
  Scope1 : Scope  NumInputPorts=3
  Sum : Sum  Inputs=|++
  kinematics from Euler angles : Subsystem
  rigid-body dynamics : Subsystem
  eta : Outport
  wires:
  kinematics from Euler angles/1(eta) -> eta/1, Gravity/1(eta_euler), Scope1/3
  tau_p/1 -> Sum/1  "tau_p"
  Sum/1 -> Scope1/1, rigid-body dynamics/1(tau)  "tau"
  rigid-body dynamics/1(nu_subsystem) -> Scope1/2, kinematics from Euler angles/1(nu)
  Gravity/1(tau_g) -> Sum/2
  x_0/1 -> kinematics from Euler angles/2(x_0)

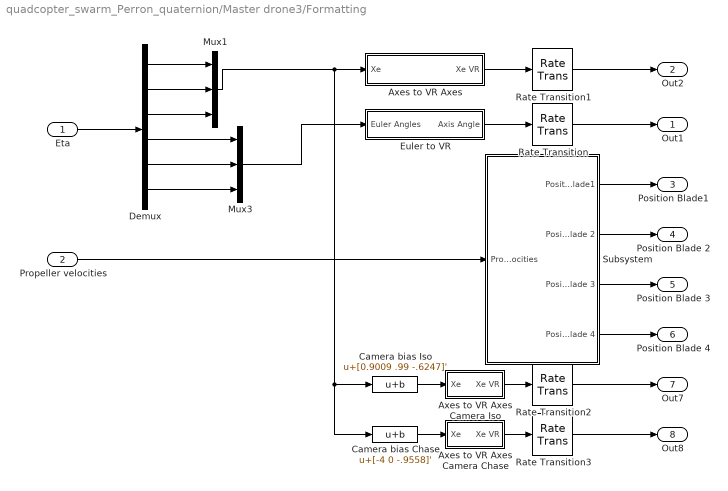
== system quadcopter_swarm_Perron_quaternion/Master drone3/Formatting ==
  Eta : Inport
  Propeller velocities : Inport  Port=2
  Axes to VR Axes : Subsystem
  Axes to VR Axes Camera Chase : Subsystem
  Axes to VR Axes Camera Iso : Subsystem
  Camera bias Chase : Bias  Bias=[-4 0 -.9558]'  SaturateOnIntegerOverflow=off
  Camera bias Iso : Bias  Bias=[0.9009 .99 -.6247]'  SaturateOnIntegerOverflow=off
  Demux : Demux  Outputs=6
  Euler to VR : Subsystem
  Mux1 : Mux  Inputs=3
  Mux3 : Mux  Inputs=3
  Rate Transition{,1..3} (4 alike) : RateTransition
  Subsystem : Subsystem
  Out1 : Outport
  Out2 : Outport  Port=2
  Position Blade1 : Outport  Port=3
  Position Blade 2 : Outport  Port=4
  Position Blade 3 : Outport  Port=5
  Position Blade 4 : Outport  Port=6
  Out7 : Outport  Port=7
  Out8 : Outport  Port=8
  wires:
  Rate Transition2/1 -> Out7/1
  Propeller velocities/1 -> Subsystem/1(Propeller velocities)
  Subsystem/3(Position Blade 3) -> Position Blade 3/1
  Subsystem/1(Position Blade1) -> Position Blade1/1
  Mux3/1 -> Euler to VR/1(Euler Angles)
  Camera bias Chase/1 -> Axes to VR Axes Camera Chase/1(Xe)
  Axes to VR Axes Camera Chase/1(Xe VR) -> Rate Transition3/1
  Subsystem/2(Position Blade 2) -> Position Blade 2/1
  Axes to VR Axes Camera Iso/1(Xe VR) -> Rate Transition2/1
  Euler to VR/1(Axis Angle) -> Rate Transition/1
  Axes to VR Axes/1(Xe VR) -> Rate Transition1/1
  Rate Transition1/1 -> Out2/1
  Camera bias Iso/1 -> Axes to VR Axes Camera Iso/1(Xe)
  Mux1/1 -> Camera bias Chase/1, Camera bias Iso/1, Axes to VR Axes/1(Xe)
  Rate Transition3/1 -> Out8/1
  Rate Transition/1 -> Out1/1
  Subsystem/4(Position Blade 4) -> Position Blade 4/1
  Demux/2 -> Mux1/2
  Demux/5 -> Mux3/2
  Demux/3 -> Mux1/3
  Eta/1 -> Demux/1
  Demux/1 -> Mux1/1
  Demux/4 -> Mux3/1
  Demux/6 -> Mux3/3

== system quadcopter_swarm_Perron_quaternion/Master drone3/PID controllers ==
  position ref : Inport
  eta : Inport  Port=2
  Inner-loop controllers : Subsystem
  Manual Switch : ManualSwitch
  Pad3 : dspsigops/Pad  padAlong=Rows  dimsToPad=1  valSrc=Specify via dialog  padVal=0  spec=Output size  padNumOutRowsSpecMethod=User-specified  numOutRows=1  padNumOutColsSpecMethod=User-specified  numOutCols=6  isVarDimsMode=off  padBeginning=0  padEnd=0  outSizeMode=User-specified  outSize=1  padSigAt=Beginning  trunc_flag=None  roundingMode=Floor  overflowMode=off  truncOrWrapMode=Truncate  wrap_flag=None
  Refs (alt. + Euler angles) : Constant  Value=[-20;0;20;0]  VectorParams1D=off
  outer-loop controllers output : Scope
  outer-loop position controller : Subsystem
  tau_p : Outport
  wires:
  position ref/1 -> outer-loop position controller/1(position ref)
  outer-loop position controller/1(alt. + Euler angles) -> Manual Switch/1, outer-loop controllers output/1
  eta/1 -> Inner-loop controllers/2(eta), outer-loop position controller/2(eta_euler)  "eta_euler"
  Refs (alt. + Euler angles)/1 -> Manual Switch/2
  Manual Switch/1 -> Inner-loop controllers/1(refs)  "alt. + Euler angles"
  Pad3/1 -> tau_p/1
  Inner-loop controllers/1(Fz,mx,my,mz) -> Pad3/1

== system quadcopter_swarm_Perron_quaternion/Master drone3/Quadcopter model Euler ==
  tau_p : Inport
  x_0 : Inport  Port=2
  Gravity : Subsystem
      settings: PortSchema="{\"entries\":[{\"content\":{\"sides\":[{\"content\":{\"connectorIds\":[\"Out1\",\"In1\"]},\"type\":\"ConnectorPlacement.EquallySpacedRectSide\",\"uuid\":\"bc23a1f5-cdb9-4283-9ea4-cdee480fdcbc\"},{\"content\":{\"side\":\"RIGHT\"},\"type\":\"ConnectorPlacement.EquallySpacedRectSide\",\"uuid\":\"6d80009b-5037-4ff5-9c53-c950dec4dc37\"},{\"content\":{\"side\":\"TOP\"},\"type\":\"ConnectorPlacement.EquallySpacedRectSide\",\"uuid\":\"00364382-26ff-4cd9-a2a2-07aec872e2b0\"}]},\"type\":\"ConnectorPlacement.EquallySpacedConnector\",\"uuid\":\"88fcb791-5b95-44c0-bf21-2ced4fb8e0fb\"}],\"packageUris\":[\"http://schema.mathworks.com/mf0/Connector/R2020b\"],\"version\":\"1.0\"}"
  Scope1 : Scope  NumInputPorts=3
  Sum : Sum  Inputs=|++
  kinematics from Euler angles : Subsystem
  rigid-body dynamics : Subsystem
  eta : Outport
  wires:
  kinematics from Euler angles/1(eta) -> eta/1, Gravity/1(eta_euler), Scope1/3
  tau_p/1 -> Sum/1  "tau_p"
  Sum/1 -> Scope1/1, rigid-body dynamics/1(tau)  "tau"
  rigid-body dynamics/1(nu_subsystem) -> Scope1/2, kinematics from Euler angles/1(nu)
  Gravity/1(tau_g) -> Sum/2
  x_0/1 -> kinematics from Euler angles/2(x_0)

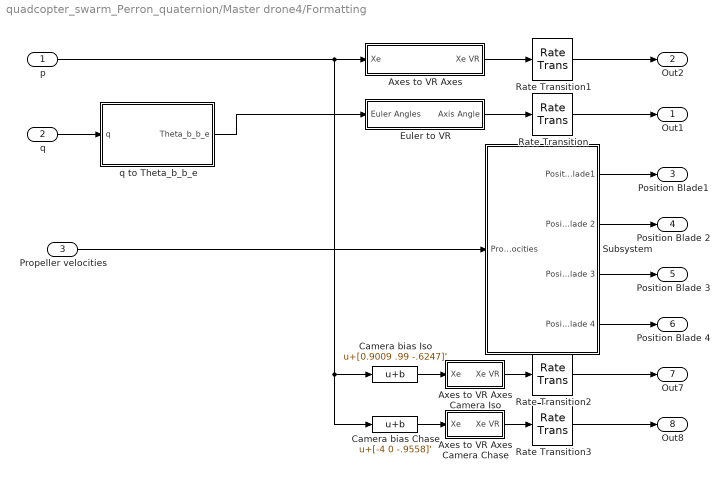
== system quadcopter_swarm_Perron_quaternion/Master drone4/Formatting ==
  p : Inport
  q : Inport  Port=2
  Propeller velocities : Inport  Port=3
  Axes to VR Axes : Subsystem
  Axes to VR Axes Camera Chase : Subsystem
  Axes to VR Axes Camera Iso : Subsystem
  Camera bias Chase : Bias  Bias=[-4 0 -.9558]'  SaturateOnIntegerOverflow=off
  Camera bias Iso : Bias  Bias=[0.9009 .99 -.6247]'  SaturateOnIntegerOverflow=off
  Euler to VR : Subsystem
  Rate Transition{,1..3} (4 alike) : RateTransition
  Subsystem : Subsystem
  q to Theta_b_b_e : Subsystem
  Out1 : Outport
  Out2 : Outport  Port=2
  Position Blade1 : Outport  Port=3
  Position Blade 2 : Outport  Port=4
  Position Blade 3 : Outport  Port=5
  Position Blade 4 : Outport  Port=6
  Out7 : Outport  Port=7
  Out8 : Outport  Port=8
  wires:
  Rate Transition2/1 -> Out7/1
  Propeller velocities/1 -> Subsystem/1(Propeller velocities)
  Subsystem/3(Position Blade 3) -> Position Blade 3/1
  Subsystem/1(Position Blade1) -> Position Blade1/1
  q to Theta_b_b_e/1(Theta_b_b_e) -> Euler to VR/1(Euler Angles)
  Camera bias Chase/1 -> Axes to VR Axes Camera Chase/1(Xe)
  Axes to VR Axes Camera Chase/1(Xe VR) -> Rate Transition3/1
  Subsystem/2(Position Blade 2) -> Position Blade 2/1
  Axes to VR Axes Camera Iso/1(Xe VR) -> Rate Transition2/1
  Euler to VR/1(Axis Angle) -> Rate Transition/1
  Axes to VR Axes/1(Xe VR) -> Rate Transition1/1
  Rate Transition1/1 -> Out2/1
  Camera bias Iso/1 -> Axes to VR Axes Camera Iso/1(Xe)
  p/1 -> Camera bias Chase/1, Camera bias Iso/1, Axes to VR Axes/1(Xe)
  Rate Transition3/1 -> Out8/1
  Rate Transition/1 -> Out1/1
  Subsystem/4(Position Blade 4) -> Position Blade 4/1
  q/1 -> q to Theta_b_b_e/1(q)
